simulink model "mtriggersubsys"  (Simulink 7.5)
settings: Solver=FixedStepDiscrete  StartTime=0.0  StopTime=10.0  FixedStep=1  RelTol=1e-3
settings Model: Creator=mtocci  LastModifiedBy=mtocci
settings DataIOCC: LimitDataPoints=off  SaveFormat=StructureWithTime
settings OptimizationCC: InlineParams=on
settings DebuggingCC: StrictBusMsg=ErrorOnBusTreatedAsVector

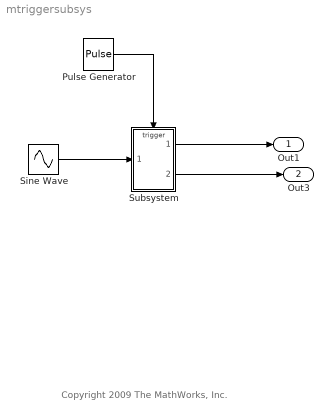
== system mtriggersubsys ==
  note: Copyright 2009 The MathWorks, Inc.
  Pulse Generator : DiscretePulseGenerator  Amplitude=[1 1 2 2]  Period=2  PulseWidth=1  PhaseDelay=0  SampleTime=1
  Sine Wave : Sin  SineType=Sample based  Amplitude=1  Bias=0  Frequency=1  Phase=0  Samples=5  SampleTime=1  Offset=0
  Subsystem : Subsystem
  Out1 : Outport  OutDataType=fixdt(1, 16)  OutScaling=2^0  InitialOutput=0
  Out3 : Outport  Port=2  OutDataType=fixdt(1, 16)  OutScaling=2^0  InitialOutput=0
  wires:
  Subsystem/1(Out1) -> Out1/1
  Subsystem/2(Out3) -> Out3/1
  Sine Wave/1 -> Subsystem/1(In2)
  Pulse Generator/1 -> Subsystem/Trigger

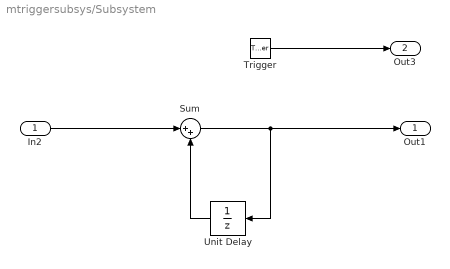
== system mtriggersubsys/Subsystem ==
  In2 : Inport  OutDataType=fixdt(1, 16)  OutScaling=2^0
  Trigger : TriggerPort  ShowOutputPort=on  OutputDataType=int8
  Sum : Sum  Inputs=|++  OutDataType=fixdt(1, 16)  OutScaling=2^0
  Unit Delay : UnitDelay  SampleTime=-1
  Out1 : Outport  OutDataType=fixdt(1, 16)  OutScaling=2^0  InitialOutput=0
  Out3 : Outport  Port=2  OutDataType=fixdt(1, 16)  OutScaling=2^0  InitialOutput=0
  wires:
  In2/1 -> Sum/1
  Sum/1 -> Out1/1, Unit Delay/1
  Unit Delay/1 -> Sum/2
  Trigger/1 -> Out3/1
